simulink model "simulinkforTests"  (R2017b)
settings: Solver=ode45  StartTime=0.0  StopTime=300  RelTol=1e-3  EnableMultiTasking=on
libraries: fuzblock x1
settings Model: ModifiedComment=Vian -- Sat Nov 25 19:55:49 2017 -- Version 1.34  Creator=Serafim  LastModifiedBy=Vian
settings Model: ModifiedHistory=|
  | Vian -- Sat Nov 25 19:49:10 2017 -- Version 1.33
  | 
  | Vian -- Sat Nov 25 19:47:05 2017 -- Version 1.32
  | 
  | Vian -- Sat Nov 25 19:46:08 2017 -- Version 1.31
  | 
  | Vian -- Sat Nov 25 19:45:57 2017 -- Version 1.30
settings SolverCC: ZeroCrossControl=DisableAll
settings DataIOCC: LimitDataPoints=on  SaveFormat=Array  SignalLoggingSaveFormat=ModelDataLogs
settings OptimizationCC: LifeSpan=inf
settings DebuggingCC: UnderspecifiedInitializationDetection=Classic  MergeDetectMultiDrivingBlocksExec=none  SolverPrmCheckMsg=warning  MultiTaskDSMMsg=warning  MultiTaskCondExecSysMsg=none  StateNameClashWarn=warning  StrictBusMsg=None  SFUnexpectedBacktrackingDiag=warning  SFNoUnconditionalDefaultTransitionDiag=warning  SFExecutionAtInitializationDiag=none
settings HardwareCC: ProdBitPerPointer=32  ProdBitPerSizeT=32  ProdBitPerPtrDiffT=32  ProdLargestAtomicFloat=None  ProdIntDivRoundTo=Undefined  ProdEndianess=Unspecified  ProdWordSize=32  ProdHWDeviceType=32-bit Generic
settings ModelReferenceCC: PropagateSignalLabelsOutOfModel=off
settings CodeAppCC: StateflowObjectComments=on
settings GRTTargetCC: TargetLangStandard=C89/C90 (ANSI)  GeneratePreprocessorConditionals=Disable all
settings ConfigComp: CovMetricSettings=dw  CovHtmlReporting=on  CovSaveCumulativeToWorkspaceVar=on  CovSaveSingleToWorkspaceVar=on  CovExternalEMLEnable=off  CovSFcnEnable=off

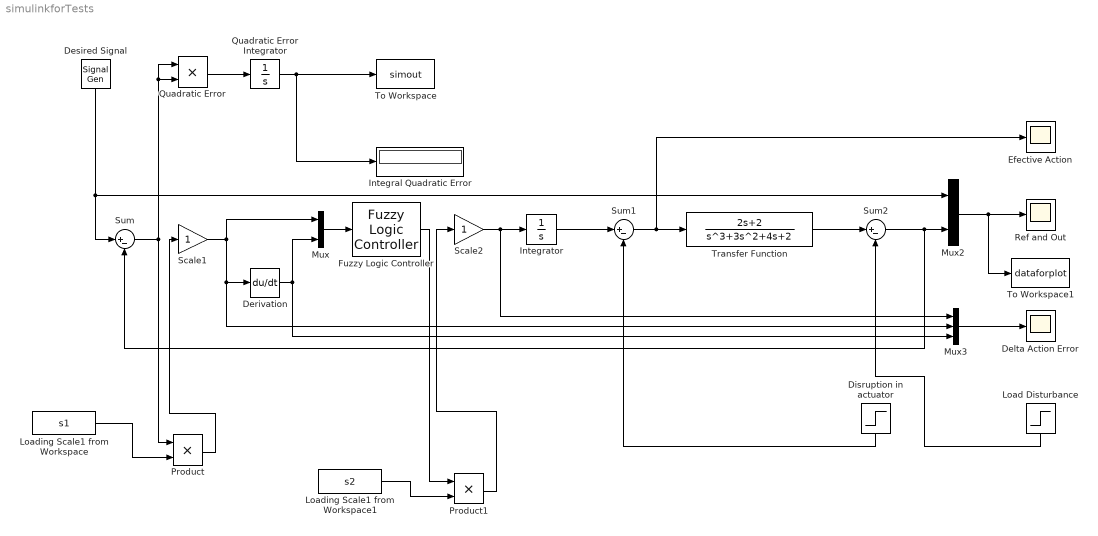
== system simulinkforTests ==
  "                               Load Disturbance   " : Step  Time=225  After=0  SampleTime=0
  Delta Action Error : Scope
  Derivation : Derivative
  "Desired Signal   " : SignalGenerator  Frequency=0.01
  "Disruption in actuator     " : Step  Time=125  After=0  SampleTime=0
  "Efective Action " : Scope
  Fuzzy Logic Controller : fuzblock/Fuzzy Logic  Controller  FIS='Fuzzy.fis'  OutputSampleNumber=101  DataType=double  FuzzifiedInputs=off  RuleFiringStrengths=off  RuleOutputs=off  AggregatedOutputs=off  SimulateUsing=Interpreted execution
  Integral Quadratic Error : Display
  "Integrator " : Integrator
  Loading Scale1 from Workspace : FromWorkspace  VariableName=s1  SampleTime=0
  Loading Scale1 from Workspace1 : FromWorkspace  VariableName=s2  SampleTime=0
  Mux : Mux  Inputs=2
  Mux2 : Mux  Inputs=2
  Mux3 : Mux  Inputs=3
  Product : Product
  Product1 : Product
  "Quadratic Error " : Product
  "Quadratic Error Integrator " : Integrator
  Ref and Out : Scope
  Scale1 : Gain
  Scale2 : Gain
  Sum : Sum  Inputs=|+-
  Sum1 : Sum  Inputs=|+-
  Sum2 : Sum  Inputs=|+-
  To Workspace : ToWorkspace  VariableName=simout  SaveFormat=Timeseries  SampleTime=-1
  To Workspace1 : ToWorkspace  VariableName=dataforplot  SaveFormat=Timeseries  SampleTime=-1
  Transfer Function : TransferFcn  Numerator=[2 2]  Denominator=[1 3 4 2]
  wires:
  "Desired Signal   "/1 -> Sum/1, Mux2/1
  Sum/1 -> Product/1, "Quadratic Error "/1, "Quadratic Error "/2
  Scale1/1 -> Mux3/2, Derivation/1, Mux/1
  "Quadratic Error "/1 -> "Quadratic Error Integrator "/1
  "Quadratic Error Integrator "/1 -> Integral Quadratic Error/1, To Workspace/1
  Derivation/1 -> Mux3/3, Mux/2
  Mux/1 -> Fuzzy Logic Controller/1
  Fuzzy Logic Controller/1 -> Product1/1
  Scale2/1 -> Mux3/1, "Integrator "/1
  "Integrator "/1 -> Sum1/1
  Sum1/1 -> "Efective Action "/1, Transfer Function/1
  Transfer Function/1 -> Sum2/1
  Sum2/1 -> Sum/2, Mux2/2
  Mux2/1 -> To Workspace1/1, Ref and Out/1
  Mux3/1 -> Delta Action Error/1
  "                               Load Disturbance   "/1 -> Sum2/2
  "Disruption in actuator     "/1 -> Sum1/2
  Loading Scale1 from Workspace/1 -> Product/2
  Product/1 -> Scale1/1
  Loading Scale1 from Workspace1/1 -> Product1/2
  Product1/1 -> Scale2/1
